simulink model "SGN_sim"  (R2024a)
settings: Solver=FixedStepDiscrete  StartTime=0.0  StopTime=time(end)  RelTol=1e-3
values from neighbouring files (symbols this model uses):
  B_n = B_n*1e-3    [init_sim.m]
  bias_gyro = 0.5*(pi/180)*[1 1 1]'    [init_sim.m]
  f_mag = 50    [init_sim.m]
  g_n = [ 0 0 g ]'    [init_sim.m]
  P0_att = [Cov_quat*eye(4), zeros(4,3); zeros(3,4), Cov_omega_bias*eye(3)]    [init_sim.m]
  P0_pv = diag([Cov_pos Cov_pos Cov_pos Cov_vel Cov_vel Cov_vel])    [init_sim.m]
  Points = sf*[ 0   0  0 ... (first row only)    [init_sim.m]
  pos_0 = tmd(1,2:4)'    [init_sim.m]
  quat_0 = quat_c(1,:)'    [init_sim.m]
  ST = 1/100    (= 0.01)    [traj_gen.m]
  Var_acc = (g*12e-6)^2*(1/ST)    [init_sim.m]
  Var_gyro = (0.014*pi/180)^2*(1/ST)    [init_sim.m]
  Var_mag = (40e-3)^2*f_mag    (= 0.08)    [init_sim.m]
  Var_uwb = 0.1^2    (= 0.01)    [init_sim.m]
  vel_0 = [0 0 0]'    [init_sim.m]
  vel_0_t = vel_n(1,:)'    [init_sim.m]
undefined symbols (not defined in the file or in its folder): DiscIntNeverNeededParam
settings Model: Creator=gigan  LastModifiedBy=gigan

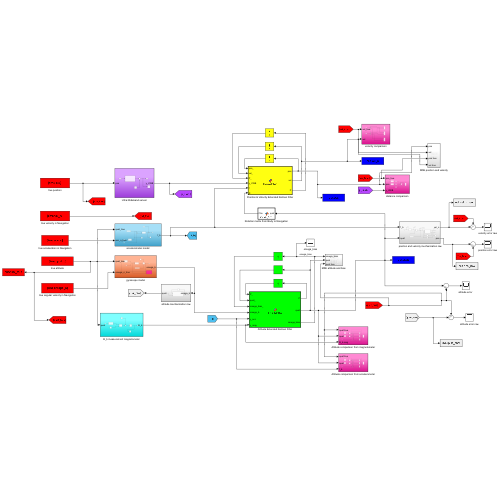
[thumbnail: Simulink's stored preview of the top-level diagram]
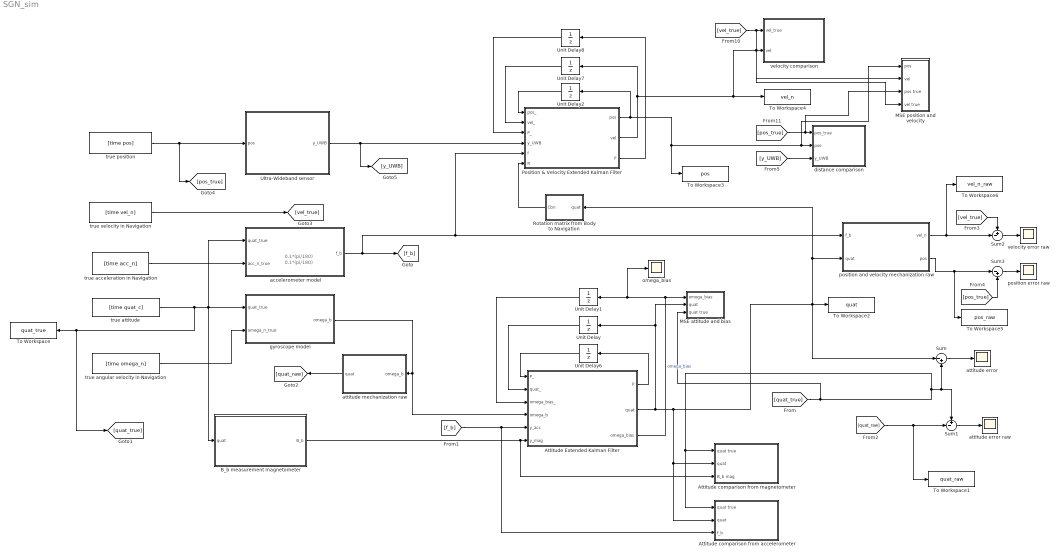
== system SGN_sim ==
  note: 0.1*(pi/180)
  note: 0.1*(pi/180)
  " position and velocity mechanization raw" : Subsystem
  Attitude Extended Kalman Filter : MATLAB Function  TreatAsAtomicUnit=on
  Attitude comparison from accelerometer : Subsystem
  Attitude comparison from magnetometer : Subsystem
  B_b measurement magnetometer : Subsystem
  MSE attitude and bias : Subsystem
  MSE position and velocity : Subsystem
  Position & Velocity Extended Kalman Filter : MATLAB Function  TreatAsAtomicUnit=on
  Rotation matrix from Body to Navigation : MATLAB Function  TreatAsAtomicUnit=on
  Sum : Sum  Inputs=|-+
  Sum1 : Sum  Inputs=+-|
  Sum2 : Sum  Inputs=+-|
  Sum3 : Sum  Inputs=|-+
  To Workspace : ToWorkspace  VariableName=quat_true  SaveFormat=Timeseries  SampleTime=-1
  To Workspace1 : ToWorkspace  VariableName=quat_raw  SaveFormat=Timeseries  SampleTime=-1
  To Workspace2 : ToWorkspace  VariableName=quat  SaveFormat=Timeseries  SampleTime=-1
  To Workspace3 : ToWorkspace  VariableName=pos  SaveFormat=Timeseries  SampleTime=-1
  To Workspace4 : ToWorkspace  VariableName=vel_n  SaveFormat=Timeseries  SampleTime=-1
  To Workspace5 : ToWorkspace  VariableName=pos_raw  SaveFormat=Timeseries  SampleTime=-1
  To Workspace6 : ToWorkspace  VariableName=vel_n_raw  SaveFormat=Timeseries  SampleTime=-1
  Ultra-Wideband sensor : Subsystem
  Unit Delay : UnitDelay  InitialCondition=quat_0  SampleTime=-1  HasFrameUpgradeWarning=on
  Unit Delay1 : UnitDelay  InitialCondition=[0 0 0]'  SampleTime=-1  HasFrameUpgradeWarning=on
  Unit Delay2 : UnitDelay  InitialCondition=pos_0  SampleTime=-1  HasFrameUpgradeWarning=on
  Unit Delay6 : UnitDelay  InitialCondition=P0_att  SampleTime=-1  HasFrameUpgradeWarning=on
  Unit Delay7 : UnitDelay  InitialCondition=vel_0  SampleTime=-1  HasFrameUpgradeWarning=on
  Unit Delay8 : UnitDelay  InitialCondition=P0_pv  SampleTime=-1  HasFrameUpgradeWarning=on
  accelerometer model : Subsystem
  "attitude error " : Scope
  attitude error raw : Scope
  attitude mechanization raw : Subsystem
  distance comparison : Subsystem
  gyroscope model : Subsystem
  omega_bias : Scope
  position error raw : Scope
  true acceleration in Navigation : FromWorkspace  VariableName=[time acc_n]
  true angular velocity in Navigation : FromWorkspace  VariableName=[time omega_n]
  true attitude : FromWorkspace  VariableName=[time quat_c]
  true position : FromWorkspace  VariableName=[time pos]
  true velocity in Navigation : FromWorkspace  VariableName=[time vel_n]
  velocity comparison : Subsystem
  velocity error raw : Scope
  wires:
  true attitude/1 -> To Workspace/1, [quat_true], gyroscope model/1(quat_true), accelerometer model/1(quat_true), B_b measurement magnetometer/1(quat)
  true angular velocity in Navigation/1 -> gyroscope model/2(omega_n_true)
  true acceleration in Navigation/1 -> accelerometer model/2(acc_n_true)
  accelerometer model/1(f_b) -> [f_b], " position and velocity mechanization raw"/1(f_b), Position & Velocity Extended Kalman Filter/5(f)
  gyroscope model/1(omega_b) -> Attitude Extended Kalman Filter/4(omega_b), attitude mechanization raw/1(omega_b)
  attitude mechanization raw/1(quat) -> [quat_raw]
  [quat_true] -> MSE attitude and bias/3(quat true), Attitude comparison from accelerometer/1(quat true), Attitude comparison from magnetometer/1(quat true), Sum1/1, Sum/2
  Sum/1 -> "attitude error "/1
  Sum1/1 -> attitude error raw/1
  [quat_raw] -> Sum1/2, To Workspace1/1
  " position and velocity mechanization raw"/1(vel_n) -> To Workspace6/1, Sum2/2
  " position and velocity mechanization raw"/2(pos) -> Sum3/1, To Workspace5/1
  Sum2/1 -> velocity error raw/1
  Sum3/1 -> position error raw/1
  true position/1 -> [pos_true], Ultra-Wideband sensor/1(pos)
  true velocity in Navigation/1 -> [vel_true]
  [vel_true] -> Sum2/1
  [pos_true] -> Sum3/2
  Attitude Extended Kalman Filter/1(P) -> Unit Delay6/1
  Unit Delay6/1 -> Attitude Extended Kalman Filter/1(P_)
  Unit Delay/1 -> Attitude Extended Kalman Filter/2(quat_)
  Attitude Extended Kalman Filter/3(omega_bias) -> MSE attitude and bias/1(omega_bias), omega_bias/1, Unit Delay1/1  "omega_bias"
  B_b measurement magnetometer/1(B_b) -> Attitude comparison from magnetometer/3(B_b mag), Attitude Extended Kalman Filter/6(y_mag)
  Attitude Extended Kalman Filter/2(quat) -> Attitude comparison from magnetometer/2(quat), Attitude comparison from accelerometer/2(quat), Sum/1, To Workspace2/1, Rotation matrix from Body to Navigation/1(quat), " position and velocity mechanization raw"/2(quat), MSE attitude and bias/2(quat), Unit Delay/1
  [f_b] -> Attitude comparison from accelerometer/3("f_b "), Attitude Extended Kalman Filter/5(y_acc)
  Unit Delay1/1 -> Attitude Extended Kalman Filter/3(omega_bias_)
  [pos_true] -> MSE position and velocity/3(pos true), distance comparison/1(pos_true)
  [vel_true] -> MSE position and velocity/4(vel true), velocity comparison/1(vel_true)
  Position & Velocity Extended Kalman Filter/1(pos) -> To Workspace3/1, MSE position and velocity/1(pos), distance comparison/2(pos), Unit Delay2/1
  Position & Velocity Extended Kalman Filter/3(P) -> Unit Delay8/1
  Position & Velocity Extended Kalman Filter/2(vel) -> Unit Delay7/1, MSE position and velocity/2(vel), velocity comparison/2(vel), To Workspace4/1
  Unit Delay2/1 -> Position & Velocity Extended Kalman Filter/1(pos_)
  Ultra-Wideband sensor/1(y_UWB) -> [y_UWB], Position & Velocity Extended Kalman Filter/4(y_UWB)
  Unit Delay7/1 -> Position & Velocity Extended Kalman Filter/2(vel_)
  Unit Delay8/1 -> Position & Velocity Extended Kalman Filter/3(P_)
  [y_UWB] -> distance comparison/3(y_UWB)
  Rotation matrix from Body to Navigation/1(Cbn) -> Position & Velocity Extended Kalman Filter/6(R)

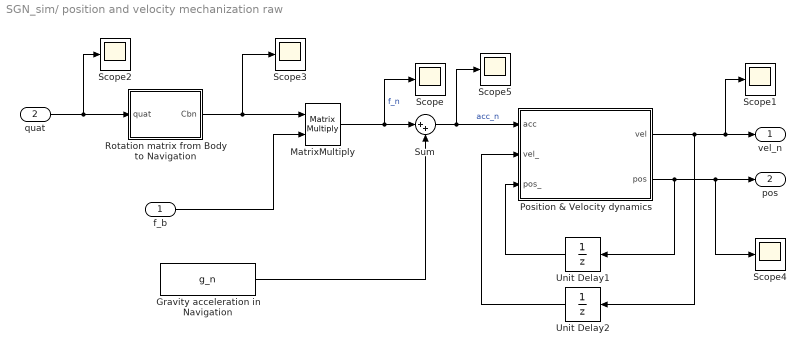
== system SGN_sim/ position and velocity mechanization raw ==
  f_b : Inport
  quat : Inport  Port=2
  Gravity acceleration in Navigation : Constant  Value=g_n
  MatrixMultiply : Product  Multiplication=Matrix(*)
  Position & Velocity dynamics : MATLAB Function  TreatAsAtomicUnit=on
  Rotation matrix from Body to Navigation : MATLAB Function  TreatAsAtomicUnit=on
  Scope{,1..5} (6 alike) : Scope
  Sum : Sum  Inputs=|++
  Unit Delay1 : UnitDelay  InitialCondition=pos_0  SampleTime=-1  HasFrameUpgradeWarning=on
  Unit Delay2 : UnitDelay  InitialCondition=vel_0_t  SampleTime=-1  HasFrameUpgradeWarning=on
  vel_n : Outport
  pos : Outport  Port=2
  wires:
  Rotation matrix from Body to Navigation/1(Cbn) -> MatrixMultiply/1, Scope3/1
  Position & Velocity dynamics/2(pos) -> Unit Delay1/1, Scope4/1, pos/1
  Position & Velocity dynamics/1(vel) -> Unit Delay2/1, Scope1/1, vel_n/1
  Unit Delay1/1 -> Position & Velocity dynamics/3(pos_)
  Unit Delay2/1 -> Position & Velocity dynamics/2(vel_)
  MatrixMultiply/1 -> Sum/1, Scope/1  "f_n"
  quat/1 -> Scope2/1, Rotation matrix from Body to Navigation/1(quat)
  Gravity acceleration in Navigation/1 -> Sum/2
  f_b/1 -> MatrixMultiply/2
  Sum/1 -> Scope5/1, Position & Velocity dynamics/1(acc)  "acc_n"

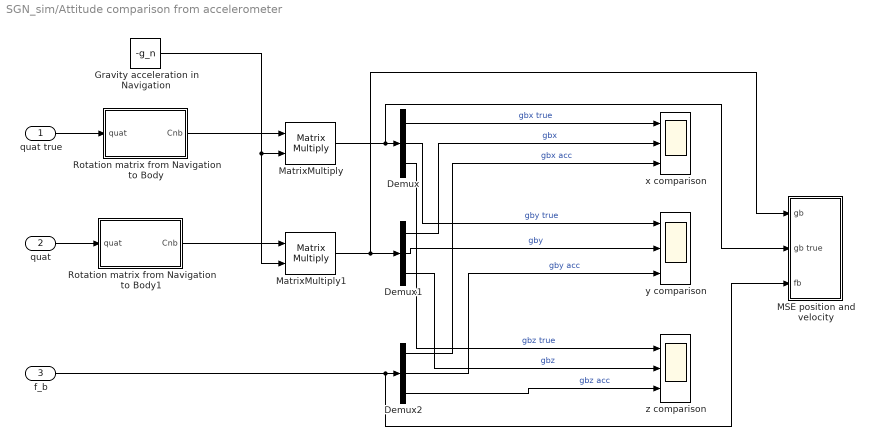
== system SGN_sim/Attitude comparison from accelerometer ==
  quat true : Inport
  quat : Inport  Port=2
  "f_b " : Inport  Port=3
  Demux : Demux  Outputs=3
  Demux1 : Demux  Outputs=3
  Demux2 : Demux  Outputs=3
  Gravity acceleration in Navigation : Constant  Value=-g_n
  MSE position and velocity : Subsystem
  MatrixMultiply : Product  Multiplication=Matrix(*)
  MatrixMultiply1 : Product  Multiplication=Matrix(*)
  Rotation matrix from Navigation to Body : MATLAB Function  TreatAsAtomicUnit=on
  Rotation matrix from Navigation to Body1 : MATLAB Function  TreatAsAtomicUnit=on
  x comparison : Scope  NumInputPorts=3
  y comparison : Scope  NumInputPorts=3
  z comparison : Scope  NumInputPorts=3
  wires:
  Demux1/1 -> x comparison/2  "gbx"
  Demux/2 -> y comparison/1  "gby true"
  "f_b "/1 -> MSE position and velocity/3(fb), Demux2/1
  MatrixMultiply/1 -> MSE position and velocity/2(gb true), Demux/1
  Demux2/1 -> x comparison/3  "gbx acc"
  Demux2/2 -> y comparison/3  "gby acc"
  Demux2/3 -> z comparison/3  "gbz acc"
  Demux1/3 -> z comparison/2  "gbz"
  MatrixMultiply1/1 -> Demux1/1, MSE position and velocity/1("gb ")
  Demux/1 -> x comparison/1  "gbx true"
  Demux1/2 -> y comparison/2  "gby"
  Demux/3 -> z comparison/1  "gbz true"
  Rotation matrix from Navigation to Body1/1(Cnb) -> MatrixMultiply1/1
  quat/1 -> Rotation matrix from Navigation to Body1/1(quat)
  quat true/1 -> Rotation matrix from Navigation to Body/1(quat)
  Rotation matrix from Navigation to Body/1(Cnb) -> MatrixMultiply/1
  Gravity acceleration in Navigation/1 -> MatrixMultiply/2, MatrixMultiply1/2

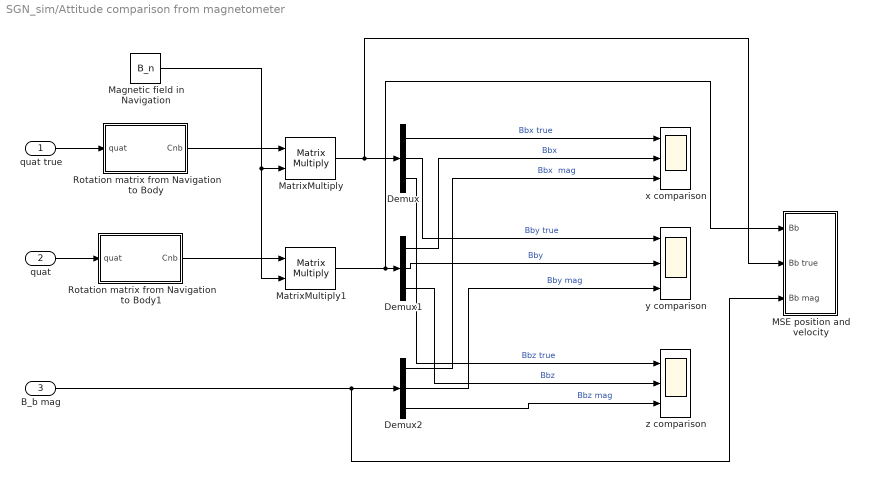
== system SGN_sim/Attitude comparison from magnetometer ==
  quat true : Inport
  quat : Inport  Port=2
  B_b mag : Inport  Port=3
  Demux : Demux  Outputs=3
  Demux1 : Demux  Outputs=3
  Demux2 : Demux  Outputs=3
  MSE position and velocity : Subsystem
  Magnetic field in Navigation : Constant  Value=B_n
  MatrixMultiply : Product  Multiplication=Matrix(*)
  MatrixMultiply1 : Product  Multiplication=Matrix(*)
  Rotation matrix from Navigation to Body : MATLAB Function  TreatAsAtomicUnit=on
  Rotation matrix from Navigation to Body1 : MATLAB Function  TreatAsAtomicUnit=on
  x comparison : Scope  NumInputPorts=3
  y comparison : Scope  NumInputPorts=3
  z comparison : Scope  NumInputPorts=3
  wires:
  Magnetic field in Navigation/1 -> MatrixMultiply1/2, MatrixMultiply/2
  Rotation matrix from Navigation to Body/1(Cnb) -> MatrixMultiply/1
  quat true/1 -> Rotation matrix from Navigation to Body/1(quat)
  quat/1 -> Rotation matrix from Navigation to Body1/1(quat)
  Rotation matrix from Navigation to Body1/1(Cnb) -> MatrixMultiply1/1
  Demux/3 -> z comparison/1  "Bbz true"
  Demux1/2 -> y comparison/2  "Bby"
  Demux/1 -> x comparison/1  "Bbx true"
  MatrixMultiply1/1 -> MSE position and velocity/1("Bb "), Demux1/1
  Demux1/3 -> z comparison/2  "Bbz"
  Demux2/3 -> z comparison/3  "Bbz mag"
  Demux2/2 -> y comparison/3  "Bby mag"
  Demux2/1 -> x comparison/3  "Bbx  mag"
  MatrixMultiply/1 -> Demux/1, MSE position and velocity/2(Bb true)
  B_b mag/1 -> MSE position and velocity/3(Bb mag), Demux2/1
  Demux/2 -> y comparison/1  "Bby true"
  Demux1/1 -> x comparison/2  "Bbx"

== system SGN_sim/B_b measurement magnetometer ==
  quat : Inport
  Magnetic field in Navigation : Constant  Value=B_n
  Magnetometer white noise : RandomNumber  Variance=Var_mag  Seed=456  SampleTime=0.1
  MatrixMultiply : Product  Multiplication=Matrix(*)
  Rate Transition : RateTransition  OutPortSampleTime=1/f_mag
  Rotation matrix from Navigation to Body : MATLAB Function  TreatAsAtomicUnit=on
  Scope : Scope
  Sum : Sum  Inputs=++|
  B_b : Outport
  wires:
  quat/1 -> Rotation matrix from Navigation to Body/1(quat)
  Rotation matrix from Navigation to Body/1(Cnb) -> MatrixMultiply/1
  Magnetic field in Navigation/1 -> MatrixMultiply/2
  Magnetometer white noise/1 -> Sum/1
  MatrixMultiply/1 -> Sum/2
  Sum/1 -> Rate Transition/1
  Rate Transition/1 -> Scope/1, B_b/1

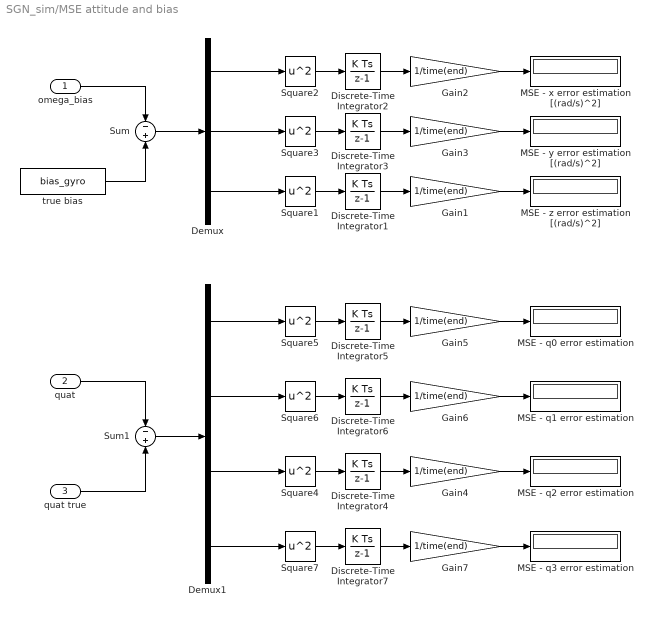
== system SGN_sim/MSE attitude and bias ==
  omega_bias : Inport
  quat : Inport  Port=2
  quat true : Inport  Port=3
  Demux : Demux  Outputs=3
  Demux1 : Demux
  Discrete-Time Integrator{1..7} (7 alike) : DiscreteIntegrator  SampleTime=-1  ICPrevOutput=DiscIntNeverNeededParam  ICPrevScaledInput=DiscIntNeverNeededParam
  Gain{1..7} (7 alike) : Gain  Gain=1/time(end)
  MSE - q0 error estimation : Display
  MSE - q1 error estimation : Display
  MSE - q2 error estimation : Display
  MSE - q3 error estimation : Display
  MSE - x error estimation [(rad/s)^2] : Display
  MSE - y error estimation [(rad/s)^2] : Display
  MSE - z error estimation [(rad/s)^2] : Display
  Square{1..7} (7 alike) : Math  Operator=square
  Sum : Sum  Inputs=-|+
  Sum1 : Sum  Inputs=-|+
  true bias : Constant  Value=bias_gyro  VectorParams1D=off
  wires:
  Discrete-Time Integrator6/1 -> Gain6/1
  Gain6/1 -> MSE - q1 error estimation/1
  Square6/1 -> Discrete-Time Integrator6/1
  Gain4/1 -> MSE - q2 error estimation/1
  Square4/1 -> Discrete-Time Integrator4/1
  Discrete-Time Integrator4/1 -> Gain4/1
  Square5/1 -> Discrete-Time Integrator5/1
  Gain5/1 -> MSE - q0 error estimation/1
  Discrete-Time Integrator5/1 -> Gain5/1
  Demux1/1 -> Square5/1
  Demux1/2 -> Square6/1
  Demux1/3 -> Square4/1
  Demux/3 -> Square1/1
  Demux/2 -> Square3/1
  Demux/1 -> Square2/1
  Discrete-Time Integrator2/1 -> Gain2/1
  Gain2/1 -> MSE - x error estimation [(rad/s)^2]/1
  Square2/1 -> Discrete-Time Integrator2/1
  Discrete-Time Integrator1/1 -> Gain1/1
  Square1/1 -> Discrete-Time Integrator1/1
  Gain1/1 -> MSE - z error estimation [(rad/s)^2]/1
  Square3/1 -> Discrete-Time Integrator3/1
  Gain3/1 -> MSE - y error estimation [(rad/s)^2]/1
  Discrete-Time Integrator3/1 -> Gain3/1
  Discrete-Time Integrator7/1 -> Gain7/1
  Square7/1 -> Discrete-Time Integrator7/1
  Gain7/1 -> MSE - q3 error estimation/1
  Demux1/4 -> Square7/1
  Sum/1 -> Demux/1
  omega_bias/1 -> Sum/1
  true bias/1 -> Sum/2
  Sum1/1 -> Demux1/1
  quat/1 -> Sum1/1
  quat true/1 -> Sum1/2

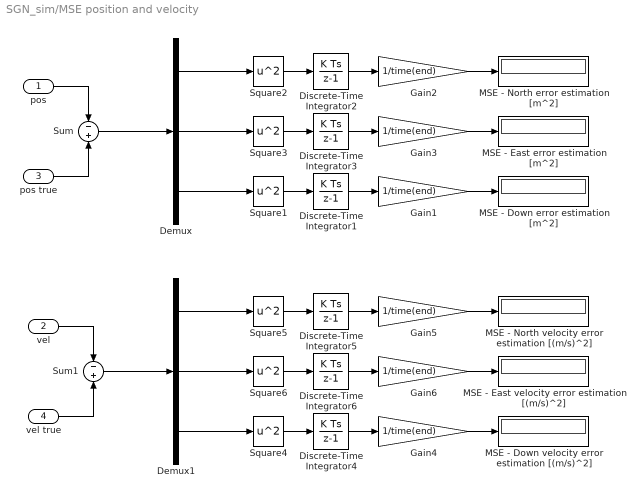
== system SGN_sim/MSE position and velocity ==
  pos : Inport
  vel : Inport  Port=2
  pos true : Inport  Port=3
  vel true : Inport  Port=4
  Demux : Demux  Outputs=3
  Demux1 : Demux  Outputs=3
  Discrete-Time Integrator{1..6} (6 alike) : DiscreteIntegrator  SampleTime=-1  ICPrevOutput=DiscIntNeverNeededParam  ICPrevScaledInput=DiscIntNeverNeededParam
  Gain{1..6} (6 alike) : Gain  Gain=1/time(end)
  MSE - Down error estimation [m^2] : Display
  MSE - Down velocity error estimation [(m/s)^2] : Display
  MSE - East error estimation [m^2] : Display
  MSE - East velocity error estimation [(m/s)^2] : Display
  MSE - North error estimation [m^2] : Display
  MSE - North velocity error estimation [(m/s)^2] : Display
  Square{1..6} (6 alike) : Math  Operator=square
  Sum : Sum  Inputs=-|+
  Sum1 : Sum  Inputs=-|+
  wires:
  Discrete-Time Integrator3/1 -> Gain3/1
  Gain3/1 -> MSE - East error estimation [m^2]/1
  Square3/1 -> Discrete-Time Integrator3/1
  Gain1/1 -> MSE - Down error estimation [m^2]/1
  Square1/1 -> Discrete-Time Integrator1/1
  Discrete-Time Integrator1/1 -> Gain1/1
  Square2/1 -> Discrete-Time Integrator2/1
  Gain2/1 -> MSE - North error estimation [m^2]/1
  Discrete-Time Integrator2/1 -> Gain2/1
  Demux/1 -> Square2/1
  Demux/2 -> Square3/1
  Demux/3 -> Square1/1
  Demux1/3 -> Square4/1
  Demux1/2 -> Square6/1
  Demux1/1 -> Square5/1
  Discrete-Time Integrator5/1 -> Gain5/1
  Gain5/1 -> MSE - North velocity error estimation [(m/s)^2]/1
  Square5/1 -> Discrete-Time Integrator5/1
  Discrete-Time Integrator4/1 -> Gain4/1
  Square4/1 -> Discrete-Time Integrator4/1
  Gain4/1 -> MSE - Down velocity error estimation [(m/s)^2]/1
  Square6/1 -> Discrete-Time Integrator6/1
  Gain6/1 -> MSE - East velocity error estimation [(m/s)^2]/1
  Discrete-Time Integrator6/1 -> Gain6/1
  pos/1 -> Sum/1
  pos true/1 -> Sum/2
  Sum/1 -> Demux/1
  vel/1 -> Sum1/1
  vel true/1 -> Sum1/2
  Sum1/1 -> Demux1/1

== system SGN_sim/Ultra-Wideband sensor ==
  pos : Inport
  Distances calculator : MATLAB Function  TreatAsAtomicUnit=on
  Scope : Scope
  Sum : Sum  Inputs=|++
  UWB white noise : RandomNumber  Variance=Var_uwb  Seed=789  SampleTime=ST
  y_UWB : Outport
  wires:
  pos/1 -> Distances calculator/1(pos)
  Distances calculator/1(d) -> Sum/1
  Sum/1 -> Scope/1, y_UWB/1
  UWB white noise/1 -> Sum/2

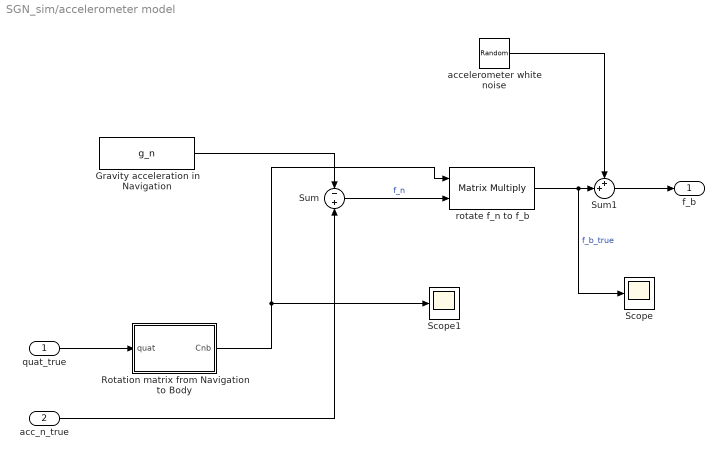
== system SGN_sim/accelerometer model ==
  quat_true : Inport
  acc_n_true : Inport  Port=2
  Gravity acceleration in Navigation : Constant  Value=g_n
  Rotation matrix from Navigation to Body : MATLAB Function  TreatAsAtomicUnit=on
  Scope : Scope
  Scope1 : Scope
  Sum : Sum  Inputs=-|+
  Sum1 : Sum  Inputs=++|
  accelerometer white noise : RandomNumber  Variance=Var_acc  Seed=123  SampleTime=ST
  rotate f_n to f_b : Product  Multiplication=Matrix(*)
  f_b : Outport
  wires:
  acc_n_true/1 -> Sum/2
  Rotation matrix from Navigation to Body/1(Cnb) -> rotate f_n to f_b/1, Scope1/1
  quat_true/1 -> Rotation matrix from Navigation to Body/1(quat)
  Sum/1 -> rotate f_n to f_b/2  "f_n"
  Gravity acceleration in Navigation/1 -> Sum/1
  rotate f_n to f_b/1 -> Scope/1, Sum1/2  "f_b_true"
  Sum1/1 -> f_b/1
  accelerometer white noise/1 -> Sum1/1

== system SGN_sim/attitude mechanization raw ==
  omega_b : Inport
  Unit Delay : UnitDelay  InitialCondition=quat_0  SampleTime=-1  HasFrameUpgradeWarning=on
  quaternion dynamics : MATLAB Function  TreatAsAtomicUnit=on
  quat : Outport
  wires:
  Unit Delay/1 -> quaternion dynamics/1(quat_)
  quaternion dynamics/1(quat) -> Unit Delay/1, quat/1
  omega_b/1 -> quaternion dynamics/2(omega_b)

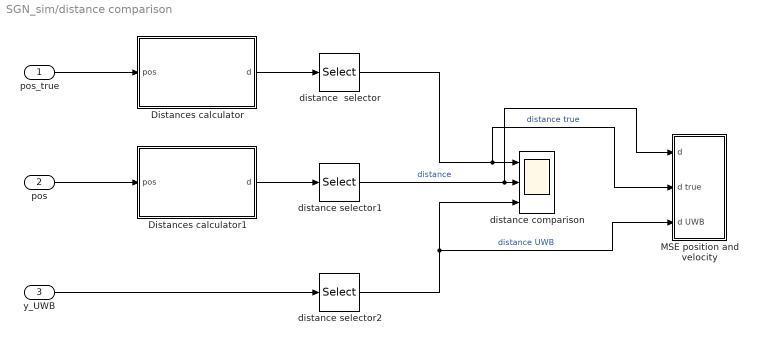
== system SGN_sim/distance comparison ==
  pos_true : Inport
  pos : Inport  Port=2
  y_UWB : Inport  Port=3
  Distances calculator : MATLAB Function  TreatAsAtomicUnit=on
  Distances calculator1 : MATLAB Function  TreatAsAtomicUnit=on
  MSE position and velocity : Subsystem
  distance  selector : Selector  InputPortWidth=6  IndexOptions=Index vector (dialog)  Indices=6  OutputSizes=1
  distance comparison : Scope  NumInputPorts=3
  distance selector1 : Selector  InputPortWidth=6  IndexOptions=Index vector (dialog)  Indices=6  OutputSizes=1
  distance selector2 : Selector  InputPortWidth=6  IndexOptions=Index vector (dialog)  Indices=6  OutputSizes=1
  wires:
  pos_true/1 -> Distances calculator/1(pos)
  pos/1 -> Distances calculator1/1(pos)
  Distances calculator/1(d) -> distance  selector/1
  Distances calculator1/1(d) -> distance selector1/1
  y_UWB/1 -> distance selector2/1
  distance selector1/1 -> MSE position and velocity/1(d), distance comparison/2  "distance"
  distance  selector/1 -> distance comparison/1, MSE position and velocity/2(d true)  "distance true"
  distance selector2/1 -> MSE position and velocity/3(d UWB), distance comparison/3  "distance UWB"

== system SGN_sim/gyroscope model ==
  quat_true : Inport
  omega_n_true : Inport  Port=2
  Add : Sum  Inputs=+++
  Rotation matrix from Navigation to Body : MATLAB Function  TreatAsAtomicUnit=on
  gyro measure vs omega_b true : Subsystem
  gyroscope bias : Constant  Value=bias_gyro  VectorParams1D=off
  gyroscope white noise : RandomNumber  Variance=Var_gyro  Seed=321  SampleTime=0.1
  rotate omega_n to omega_b : Product  Multiplication=Matrix(*)
  omega_b : Outport
  wires:
  Add/1 -> gyro measure vs omega_b true/2(omega_b), omega_b/1
  Rotation matrix from Navigation to Body/1(Cnb) -> rotate omega_n to omega_b/1
  omega_n_true/1 -> rotate omega_n to omega_b/2, gyro measure vs omega_b true/3(omega_n true)
  gyroscope bias/1 -> Add/3
  rotate omega_n to omega_b/1 -> Add/2  "omega_b_true"
  gyroscope white noise/1 -> Add/1
  quat_true/1 -> gyro measure vs omega_b true/1(quat true), Rotation matrix from Navigation to Body/1(quat)

== system SGN_sim/velocity comparison ==
  vel_true : Inport
  vel : Inport  Port=2
  Demux : Demux  Outputs=3
  Demux1 : Demux  Outputs=3
  Down comparison : Scope  NumInputPorts=2
  East comparison : Scope  NumInputPorts=2
  North comparison : Scope  NumInputPorts=2
  wires:
  Demux1/3 -> Down comparison/2  "vel down"
  Demux/3 -> Down comparison/1  "vel down true"
  Demux1/2 -> East comparison/2  "vel east"
  Demux/2 -> East comparison/1  "vel east true"
  Demux1/1 -> North comparison/2  "vel north"
  Demux/1 -> North comparison/1  "vel north true"
  vel_true/1 -> Demux/1
  vel/1 -> Demux1/1

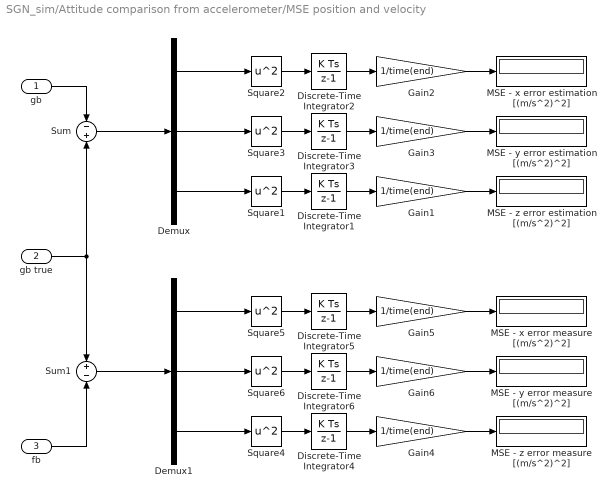
== system SGN_sim/Attitude comparison from accelerometer/MSE position and velocity ==
  "gb " : Inport
  gb true : Inport  Port=2
  fb : Inport  Port=3
  Demux : Demux  Outputs=3
  Demux1 : Demux  Outputs=3
  Discrete-Time Integrator{1..6} (6 alike) : DiscreteIntegrator  SampleTime=-1  ICPrevOutput=DiscIntNeverNeededParam  ICPrevScaledInput=DiscIntNeverNeededParam
  Gain{1..6} (6 alike) : Gain  Gain=1/time(end)
  MSE - x error estimation [(m/s^2)^2] : Display
  MSE - x error measure [(m/s^2)^2] : Display
  MSE - y error estimation [(m/s^2)^2] : Display
  MSE - y error measure [(m/s^2)^2] : Display
  MSE - z error estimation [(m/s^2)^2] : Display
  MSE - z error measure [(m/s^2)^2] : Display
  Square{1..6} (6 alike) : Math  Operator=square
  Sum : Sum  Inputs=-|+
  Sum1 : Sum  Inputs=+|-
  wires:
  Discrete-Time Integrator3/1 -> Gain3/1
  Gain3/1 -> MSE - y error estimation [(m/s^2)^2]/1
  Square3/1 -> Discrete-Time Integrator3/1
  Gain1/1 -> MSE - z error estimation [(m/s^2)^2]/1
  Square1/1 -> Discrete-Time Integrator1/1
  Discrete-Time Integrator1/1 -> Gain1/1
  Square2/1 -> Discrete-Time Integrator2/1
  Gain2/1 -> MSE - x error estimation [(m/s^2)^2]/1
  Discrete-Time Integrator2/1 -> Gain2/1
  Demux/1 -> Square2/1
  Demux/2 -> Square3/1
  Demux/3 -> Square1/1
  Demux1/3 -> Square4/1
  Demux1/2 -> Square6/1
  Demux1/1 -> Square5/1
  Discrete-Time Integrator5/1 -> Gain5/1
  Gain5/1 -> MSE - x error measure [(m/s^2)^2]/1
  Square5/1 -> Discrete-Time Integrator5/1
  Discrete-Time Integrator4/1 -> Gain4/1
  Square4/1 -> Discrete-Time Integrator4/1
  Gain4/1 -> MSE - z error measure [(m/s^2)^2]/1
  Square6/1 -> Discrete-Time Integrator6/1
  Gain6/1 -> MSE - y error measure [(m/s^2)^2]/1
  Discrete-Time Integrator6/1 -> Gain6/1
  "gb "/1 -> Sum/1
  Sum/1 -> Demux/1
  Sum1/1 -> Demux1/1
  gb true/1 -> Sum1/1, Sum/2
  fb/1 -> Sum1/2

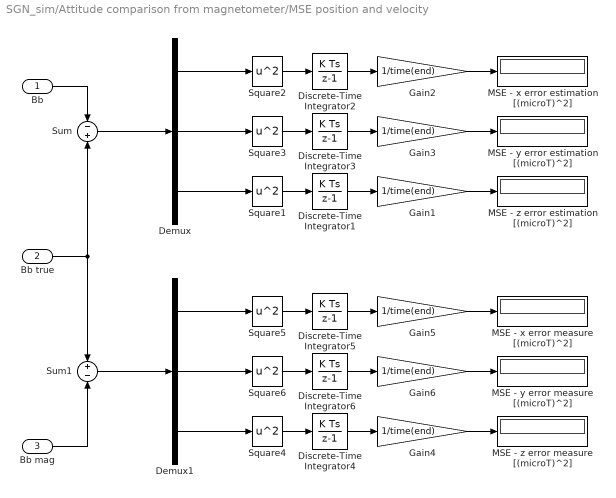
== system SGN_sim/Attitude comparison from magnetometer/MSE position and velocity ==
  "Bb " : Inport
  Bb true : Inport  Port=2
  Bb mag : Inport  Port=3
  Demux : Demux  Outputs=3
  Demux1 : Demux  Outputs=3
  Discrete-Time Integrator{1..6} (6 alike) : DiscreteIntegrator  SampleTime=-1  ICPrevOutput=DiscIntNeverNeededParam  ICPrevScaledInput=DiscIntNeverNeededParam
  Gain{1..6} (6 alike) : Gain  Gain=1/time(end)
  MSE - x error estimation [(microT)^2] : Display
  MSE - x error measure [(microT)^2] : Display
  MSE - y error estimation [(microT)^2] : Display
  MSE - y error measure [(microT)^2] : Display
  MSE - z error estimation [(microT)^2] : Display
  MSE - z error measure [(microT)^2] : Display
  Square{1..6} (6 alike) : Math  Operator=square
  Sum : Sum  Inputs=-|+
  Sum1 : Sum  Inputs=+|-
  wires:
  Discrete-Time Integrator3/1 -> Gain3/1
  Gain3/1 -> MSE - y error estimation [(microT)^2]/1
  Square3/1 -> Discrete-Time Integrator3/1
  Gain1/1 -> MSE - z error estimation [(microT)^2]/1
  Square1/1 -> Discrete-Time Integrator1/1
  Discrete-Time Integrator1/1 -> Gain1/1
  Square2/1 -> Discrete-Time Integrator2/1
  Gain2/1 -> MSE - x error estimation [(microT)^2]/1
  Discrete-Time Integrator2/1 -> Gain2/1
  Demux/1 -> Square2/1
  Demux/2 -> Square3/1
  Demux/3 -> Square1/1
  Demux1/3 -> Square4/1
  Demux1/2 -> Square6/1
  Demux1/1 -> Square5/1
  Discrete-Time Integrator5/1 -> Gain5/1
  Gain5/1 -> MSE - x error measure [(microT)^2]/1
  Square5/1 -> Discrete-Time Integrator5/1
  Discrete-Time Integrator4/1 -> Gain4/1
  Square4/1 -> Discrete-Time Integrator4/1
  Gain4/1 -> MSE - z error measure [(microT)^2]/1
  Square6/1 -> Discrete-Time Integrator6/1
  Gain6/1 -> MSE - y error measure [(microT)^2]/1
  Discrete-Time Integrator6/1 -> Gain6/1
  "Bb "/1 -> Sum/1
  Sum/1 -> Demux/1
  Sum1/1 -> Demux1/1
  Bb true/1 -> Sum1/1, Sum/2
  Bb mag/1 -> Sum1/2

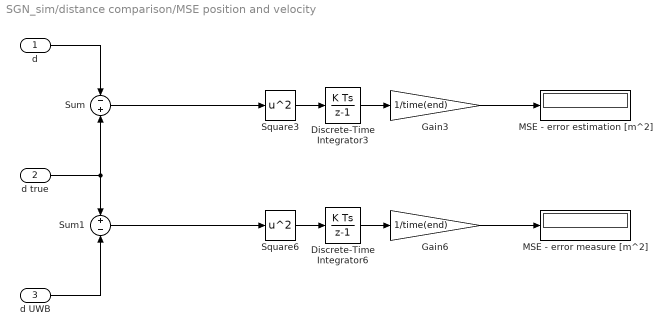
== system SGN_sim/distance comparison/MSE position and velocity ==
  d : Inport
  d true : Inport  Port=2
  d UWB : Inport  Port=3
  Discrete-Time Integrator3 : DiscreteIntegrator  SampleTime=-1  ICPrevOutput=DiscIntNeverNeededParam  ICPrevScaledInput=DiscIntNeverNeededParam
  Discrete-Time Integrator6 : DiscreteIntegrator  SampleTime=-1  ICPrevOutput=DiscIntNeverNeededParam  ICPrevScaledInput=DiscIntNeverNeededParam
  Gain3 : Gain  Gain=1/time(end)
  Gain6 : Gain  Gain=1/time(end)
  MSE - error estimation [m^2] : Display
  MSE - error measure [m^2] : Display
  Square3 : Math  Operator=square
  Square6 : Math  Operator=square
  Sum : Sum  Inputs=-|+
  Sum1 : Sum  Inputs=+|-
  wires:
  Discrete-Time Integrator3/1 -> Gain3/1
  Gain3/1 -> MSE - error estimation [m^2]/1
  Square3/1 -> Discrete-Time Integrator3/1
  Sum/1 -> Square3/1
  d/1 -> Sum/1
  d true/1 -> Sum/2, Sum1/1
  Gain6/1 -> MSE - error measure [m^2]/1
  Square6/1 -> Discrete-Time Integrator6/1
  Sum1/1 -> Square6/1
  Discrete-Time Integrator6/1 -> Gain6/1
  d UWB/1 -> Sum1/2

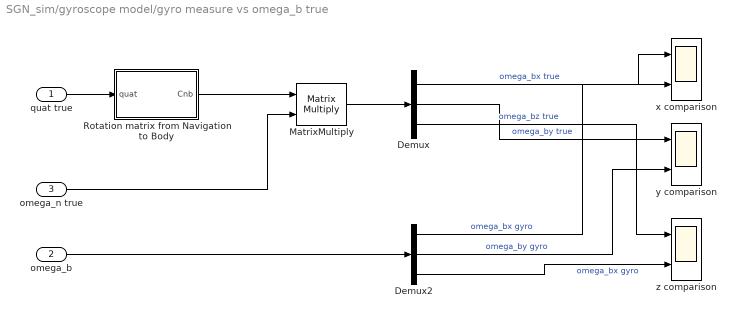
== system SGN_sim/gyroscope model/gyro measure vs omega_b true ==
  quat true : Inport
  omega_b : Inport  Port=2
  omega_n true : Inport  Port=3
  Demux : Demux  Outputs=3
  Demux2 : Demux  Outputs=3
  MatrixMultiply : Product  Multiplication=Matrix(*)
  Rotation matrix from Navigation to Body : MATLAB Function  TreatAsAtomicUnit=on
  x comparison : Scope  NumInputPorts=2
  y comparison : Scope  NumInputPorts=2
  z comparison : Scope  NumInputPorts=2
  wires:
  Rotation matrix from Navigation to Body/1(Cnb) -> MatrixMultiply/1
  quat true/1 -> Rotation matrix from Navigation to Body/1(quat)
  MatrixMultiply/1 -> Demux/1
  omega_b/1 -> Demux2/1
  omega_n true/1 -> MatrixMultiply/2
  Demux/1 -> x comparison/1  "omega_bx true"
  Demux/3 -> z comparison/1  "omega_bz true"
  Demux2/1 -> x comparison/2  "omega_bx gyro"
  Demux2/2 -> y comparison/2  "omega_by gyro"
  Demux2/3 -> z comparison/2  "omega_bx gyro"
  Demux/2 -> y comparison/1  "omega_by true"

== matlab function SGN_sim/Attitude comparison from accelerometer/Rotation matrix from Navigation to Body1 ==
  data: quat input; Cnb output
function Cnb = make_Cnb(quat)

q_w  =quat(1);
q_v = [quat(2);quat(3);quat(4)];
Q_v = [      0   -q_v(3)   q_v(2);
        q_v(3)         0  -q_v(1);
       -q_v(2)    q_v(1)        0 ];

Cnb = (q_w^2 - q_v'*q_v)*eye(3) + 2*(q_v)*q_v' + 2*q_w*Q_v;

== matlab function SGN_sim/gyroscope model/gyro measure vs omega_b true/Rotation matrix from Navigation to Body ==
  data: quat input; Cnb output
function Cnb = make_Cnb(quat)

q_w  =quat(1);
q_v = [quat(2);quat(3);quat(4)];
Q_v = [      0   -q_v(3)   q_v(2);
        q_v(3)         0  -q_v(1);
       -q_v(2)    q_v(1)        0 ];

Cnb = (q_w^2 - q_v'*q_v)*eye(3) + 2*(q_v)*q_v' + 2*q_w*Q_v;

== matlab function SGN_sim/Ultra-Wideband sensor/Distances calculator ==
  data: pos input; d output; Points parameter
function d = d_make(pos,Points)

x = pos(1); y = pos(2); z = pos(3);
d = zeros(size(Points,1),1);

for k = 1 : size(Points,1)
    d(k) = sqrt( (x - Points(k,1))^2 + (y - Points(k,2))^2 + (z - Points(k,3))^2); 
end

end

== matlab function SGN_sim/distance comparison/Distances calculator ==
  data: pos input; d output; Points parameter
function d = d_make(pos,Points)

x = pos(1); y = pos(2); z = pos(3);
d = zeros(size(Points,1),1);

for k = 1 : size(Points,1)
    d(k) = sqrt( (x - Points(k,1))^2 + (y - Points(k,2))^2 + (z - Points(k,3))^2); 
end

end

== matlab function SGN_sim/ position and velocity mechanization raw/Position & Velocity dynamics ==
  data: acc input; vel output; pos output; vel_ input; pos_ input; ST parameter
function [vel,pos] = posveldyn(acc, vel_, pos_, ST)


pos = pos_ + vel_*ST; % + 0.5*acc*ST^2;
vel = vel_ + acc*ST;

end

== matlab function SGN_sim/distance comparison/Distances calculator1 ==
  data: pos input; d output; Points parameter
function d = d_make(pos,Points)

x = pos(1); y = pos(2); z = pos(3);
d = zeros(size(Points,1),1);

for k = 1 : size(Points,1)
    d(k) = sqrt( (x - Points(k,1))^2 + (y - Points(k,2))^2 + (z - Points(k,3))^2); 
end

end

== matlab function SGN_sim/Position & Velocity Extended Kalman Filter ==
  data: pos_ input; pos output; vel_ input; P_ input; y_UWB input; f input; R input; vel output; P output; g_n parameter; ST parameter; Var_acc parameter; Var_uwb parameter; Points parameter
function [pos,vel,P] = PosVelFilter(pos_,vel_,P_,y_UWB,f,R,g_n,ST,Var_acc,Var_uwb,Points)
         [pos,vel,P] = PosVelFilter(pos_,vel_,P_,y_UWB,f,R,g_n,ST,Var_acc,Var_uwb,Points);
end

== matlab function SGN_sim/Rotation matrix from Body to Navigation ==
  data: quat input; Cbn output
function Cbn = make_Cbn(quat)

q_w  =quat(1);
q_v = [ quat(2); quat(3); quat(4) ];
Q_v = [      0   -q_v(3)   q_v(2);
        q_v(3)         0  -q_v(1);
       -q_v(2)    q_v(1)        0 ];

Cnb = (q_w^2 - q_v'*q_v)*eye(3) + 2*(q_v)*q_v' + 2*q_w*Q_v;

Cbn = Cnb';

== matlab function SGN_sim/Attitude Extended Kalman Filter ==
  data: P output; quat output; P_ input; quat_ input; omega_bias_ input; omega_b input; omega_bias output; y_acc input; y_mag input; ST parameter; g_n parameter; B_n parameter; Var_gyro parameter; Var_acc parameter; Var_mag parameter
function [P,quat,omega_bias]=AttitudeFilter(P_,quat_,omega_bias_,omega_b,y_acc,y_mag,ST, g_n, B_n,Var_gyro, Var_acc, Var_mag)
         [P,quat,omega_bias]=AttitudeFilter(P_,quat_,omega_bias_,omega_b,y_acc,y_mag,ST, g_n, B_n,Var_gyro, Var_acc, Var_mag);
end

== matlab function SGN_sim/accelerometer model/Rotation matrix from Navigation to Body ==
  data: quat input; Cnb output
function Cnb = make_Cnb(quat)

q_w  =quat(1);
q_v = [quat(2);quat(3);quat(4)];
Q_v = [      0   -q_v(3)   q_v(2);
        q_v(3)         0  -q_v(1);
       -q_v(2)    q_v(1)        0 ];

Cnb = (q_w^2 - q_v'*q_v)*eye(3) + 2*(q_v)*q_v' + 2*q_w*Q_v;

== matlab function SGN_sim/gyroscope model/Rotation matrix from Navigation to Body ==
  data: quat input; Cnb output
function Cnb = make_Cnb(quat)

q_w  =quat(1);
q_v = [quat(2);quat(3);quat(4)];
Q_v = [      0   -q_v(3)   q_v(2);
        q_v(3)         0  -q_v(1);
       -q_v(2)    q_v(1)        0 ];

Cnb = (q_w^2 - q_v'*q_v)*eye(3) + 2*(q_v)*q_v' + 2*q_w*Q_v;

== matlab function SGN_sim/Attitude comparison from magnetometer/Rotation matrix from Navigation to Body ==
  data: quat input; Cnb output
function Cnb = make_Cnb(quat)

q_w  =quat(1);
q_v = [quat(2);quat(3);quat(4)];
Q_v = [      0   -q_v(3)   q_v(2);
        q_v(3)         0  -q_v(1);
       -q_v(2)    q_v(1)        0 ];

Cnb = (q_w^2 - q_v'*q_v)*eye(3) + 2*(q_v)*q_v' + 2*q_w*Q_v;

== matlab function SGN_sim/ position and velocity mechanization raw/Rotation matrix from Body to Navigation ==
  data: quat input; Cbn output
function Cbn = make_Cbn(quat)

q_w  =quat(1);
q_v = [ quat(2); quat(3); quat(4) ];
Q_v = [      0   -q_v(3)   q_v(2);
        q_v(3)         0  -q_v(1);
       -q_v(2)    q_v(1)        0 ];

Cnb = (q_w^2 - q_v'*q_v)*eye(3) + 2*(q_v)*q_v' + 2*q_w*Q_v;

Cbn = Cnb';

== matlab function SGN_sim/Attitude comparison from magnetometer/Rotation matrix from Navigation to Body1 ==
  data: quat input; Cnb output
function Cnb = make_Cnb(quat)

q_w  =quat(1);
q_v = [quat(2);quat(3);quat(4)];
Q_v = [      0   -q_v(3)   q_v(2);
        q_v(3)         0  -q_v(1);
       -q_v(2)    q_v(1)        0 ];

Cnb = (q_w^2 - q_v'*q_v)*eye(3) + 2*(q_v)*q_v' + 2*q_w*Q_v;

== matlab function SGN_sim/Attitude comparison from accelerometer/Rotation matrix from Navigation to Body ==
  data: quat input; Cnb output
function Cnb = make_Cnb(quat)

q_w  =quat(1);
q_v = [quat(2);quat(3);quat(4)];
Q_v = [      0   -q_v(3)   q_v(2);
        q_v(3)         0  -q_v(1);
       -q_v(2)    q_v(1)        0 ];

Cnb = (q_w^2 - q_v'*q_v)*eye(3) + 2*(q_v)*q_v' + 2*q_w*Q_v;

== matlab function SGN_sim/B_b measurement magnetometer/Rotation matrix from Navigation to Body ==
  data: quat input; Cnb output
function Cnb = make_Cnb(quat)

q_w  =quat(1);
q_v = [quat(2);quat(3);quat(4)];
Q_v = [      0   -q_v(3)   q_v(2);
        q_v(3)         0  -q_v(1);
       -q_v(2)    q_v(1)        0 ];

Cnb = (q_w^2 - q_v'*q_v)*eye(3) + 2*(q_v)*q_v' + 2*q_w*Q_v;

== matlab function SGN_sim/attitude mechanization raw/quaternion dynamics ==
  data: quat_ input; quat output; omega_b input; ST parameter
function quat=quat_dynamics(quat_, omega_b,ST)

alpha = (omega_b)*ST;
alpha_norm = vecnorm(alpha);
u = alpha/alpha_norm;
quat_om = [cos(alpha_norm/2); u*sin(alpha_norm/2)];
pw=quat_(1); pv=quat_(2:4);
qw=quat_om(1); qv=quat_om(2:4);
quat=[pw*qw - (pv')*qv;
      pw*qv + qw*pv + cross(pv,qv)];
end
